simulink model "odpimp"  (Simulink 7.5)
settings: Solver=ode45  StartTime=0.0  StopTime=10.0  RelTol=1e-3
undefined symbols (not defined in the file): B, In, psien, Rt, T, Un
settings Model: Creator=Konrad  LastModifiedBy=Konrad

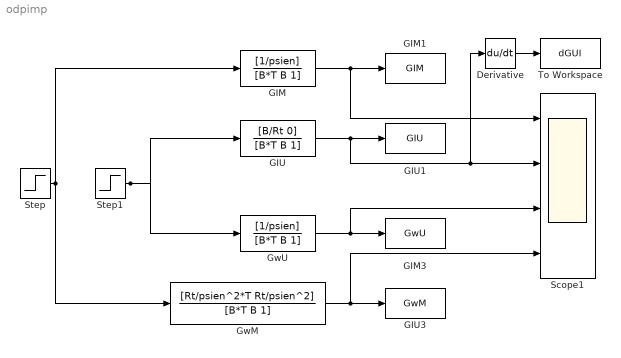
== system odpimp ==
  Derivative : Derivative
  GIM : TransferFcn  Numerator=[1/psien]  Denominator=[B*T B 1]
  GIM1 : ToWorkspace  VariableName=GIM  SampleTime=-1  SaveFormat=Structure With Time
  GIM3 : ToWorkspace  VariableName=GwU  SampleTime=-1  SaveFormat=Structure With Time
  GIU : TransferFcn  Numerator=[B/Rt 0]  Denominator=[B*T B 1]
  GIU1 : ToWorkspace  VariableName=GIU  SampleTime=-1  SaveFormat=Structure With Time
  GIU3 : ToWorkspace  VariableName=GwM  SampleTime=-1  SaveFormat=Structure With Time
  GwM : TransferFcn  Numerator=[Rt/psien^2*T Rt/psien^2]  Denominator=[B*T B 1]
  GwU : TransferFcn  Numerator=[1/psien]  Denominator=[B*T B 1]
  Scope1 : Scope  NumInputPorts=4
      settings: YMin=-5~-5~-5~-5  YMax=5~5~5~5
  Step : Step  After=psien*In  SampleTime=0
  Step1 : Step  After=Un  SampleTime=0
  To Workspace : ToWorkspace  VariableName=dGUI  SampleTime=-1  SaveFormat=Structure
  wires:
  GIM/1 -> Scope1/1, GIM1/1
  Step1/1 -> GIU/1, GwU/1
  Step/1 -> GIM/1, GwM/1
  GwU/1 -> GIM3/1, Scope1/3
  GwM/1 -> GIU3/1, Scope1/4
  Derivative/1 -> To Workspace/1
  GIU/1 -> GIU1/1, Scope1/2, Derivative/1
